simulink model "log2_float_single"  (R2018b)
settings: Solver=FixedStepDiscrete  StartTime=0.0  StopTime=1e12  RelTol=1e-3  EnableMultiTasking=on
settings Model: FPTRunName=FPA_Reference  Creator=minimales  LastModifiedBy=ekorotkyi
settings OptimizationCC: BlockReduction=off  ConditionallyExecuteInputs=off  DefaultParameterBehavior=Inlined  LifeSpan=inf
settings DebuggingCC: AlgebraicLoopMsg=error  SingleTaskRateTransMsg=error  SFUnexpectedBacktrackingDiag=warning  SFNoUnconditionalDefaultTransitionDiag=warning  SFExecutionAtInitializationDiag=none
settings HardwareCC: ProdBitPerPointer=32  ProdBitPerSizeT=32  ProdBitPerPtrDiffT=32  ProdLargestAtomicFloat=None  ProdIntDivRoundTo=Undefined  ProdEndianess=Unspecified  ProdWordSize=32  ProdHWDeviceType=ASIC/FPGA->ASIC/FPGA  ProdEqTarget=off
settings SFSimCC: SimUseLocalCustomCode=off
settings RTWCC: RTWUseLocalCustomCode=off
settings CodeAppCC: StateflowObjectComments=on
settings GRTTargetCC: TargetLangStandard=C89/C90 (ANSI)  GeneratePreprocessorConditionals=Disable all
settings ConfigComp: CovScope=Subsystem  CovPath=SIGNAL_PROCESSING_DF  CovMetricSettings=w  CovHTMLOptions=-sRT=1 -sVT=0 -aTS=1 -bRG=1 -bTC=1 -hTR=0 -nFC=0 -nFD=1 -scm=1 -bcm=1 -xEv=0 -xEM=0  CovHtmlReporting=on  CovSaveCumulativeToWorkspaceVar=on  CovSaveSingleToWorkspaceVar=on  CovExternalEMLEnable=off  CovSFcnEnable=off

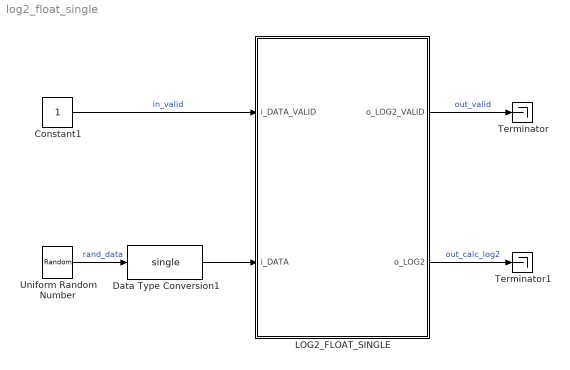
== system log2_float_single ==
  Constant1 : Constant  OutDataTypeStr=boolean  SampleTime=1
  Data Type Conversion1 : DataTypeConversion  OutDataTypeStr=single
  LOG2_FLOAT_SINGLE : Subsystem
  Terminator : Terminator
  Terminator1 : Terminator
  Uniform Random Number : UniformRandomNumber  Minimum=1  Maximum=2  SampleTime=1
  wires:
  Uniform Random Number/1 -> Data Type Conversion1/1  "rand_data"
  Constant1/1 -> LOG2_FLOAT_SINGLE/1(i_DATA_VALID)  "in_valid"
  Data Type Conversion1/1 -> LOG2_FLOAT_SINGLE/2(i_DATA)
  LOG2_FLOAT_SINGLE/1(o_LOG2_VALID) -> Terminator/1  "out_valid"
  LOG2_FLOAT_SINGLE/2(o_LOG2) -> Terminator1/1  "out_calc_log2"

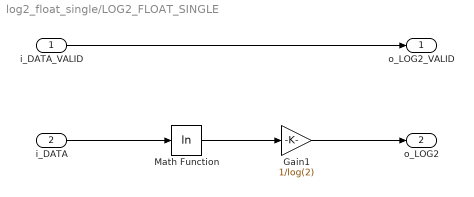
== system log2_float_single/LOG2_FLOAT_SINGLE ==
  i_DATA_VALID : Inport  OutDataTypeStr=boolean
  i_DATA : Inport  Port=2  OutDataTypeStr=single
  Gain1 : Gain  Gain=1/log(2)
  Math Function : Math  Operator=log  RndMeth=Zero  SaturateOnIntegerOverflow=on
  o_LOG2_VALID : Outport
  o_LOG2 : Outport  Port=2
  wires:
  i_DATA/1 -> Math Function/1
  Math Function/1 -> Gain1/1
  i_DATA_VALID/1 -> o_LOG2_VALID/1
  Gain1/1 -> o_LOG2/1
